simulink library "CryoDetLibCMB"  (R2016b)
settings: Solver=VariableStepAuto  StartTime=0.0  StopTime=10.0  RelTol=1e-3
values from neighbouring files (symbols this model uses):
  Fclk = Fadc    (= 307200000)    [setupCryoFPGA.m]    (also in setupCryoFPGA_CMB.m; setupCryoFPGAorig.m = 312500000)
undefined symbols (not defined in the file or in its folder): xlipgetpartsetting
libraries: xbsIndex_r4 x255, CryoDetLibCMB x19, CryoDetLib x2, simulink x1
(part 3 of 3)

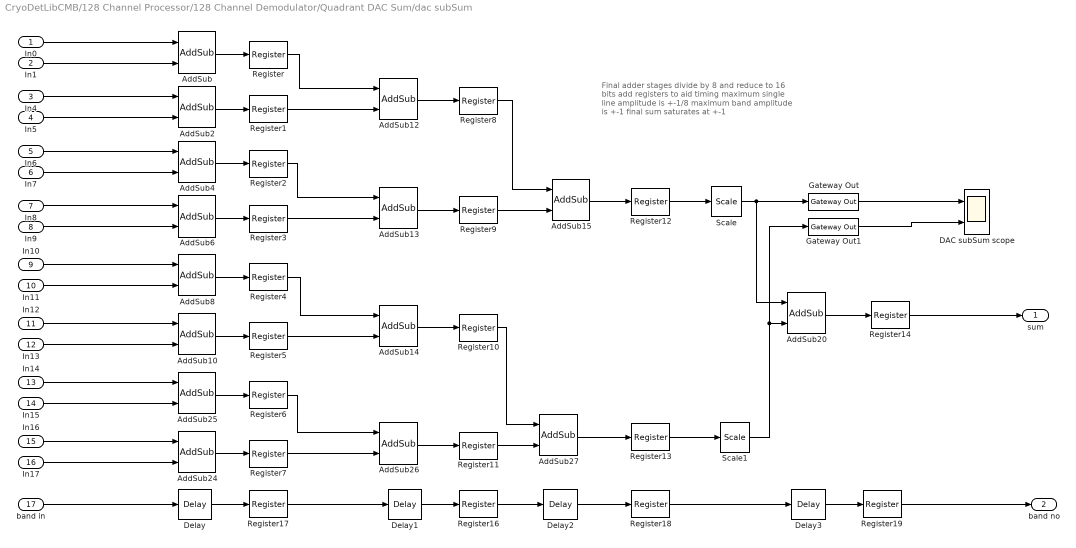
== system CryoDetLibCMB/128 Channel Processor/128 Channel Demodulator/Quadrant DAC Sum/dac subSum ==
  note: Final adder stages
      | divide by 8
      | and reduce to 16 bits
      | add registers to aid timing
      | maximum single line amplitude is +-1/8
      | maximum band amplitude is +-1
      | final sum saturates at +-1
  In0 : Inport
  In1 : Inport  Port=2
  In4 : Inport  Port=3
  In5 : Inport  Port=4
  In6 : Inport  Port=5
  In7 : Inport  Port=6
  In8 : Inport  Port=7
  In9 : Inport  Port=8
  In10 : Inport  Port=9
  In11 : Inport  Port=10
  In12 : Inport  Port=11
  In13 : Inport  Port=12
  In14 : Inport  Port=13
  In15 : Inport  Port=14
  In16 : Inport  Port=15
  In17 : Inport  Port=16
  band in : Inport  Port=17
  AddSub{,2,4,8,10,12..14,24..26} (11 alike) : xbsIndex_r4/AddSub  mode=Addition  use_carryin=off  use_carryout=off  en=off  latency=3  precision=User Defined  arith_type="Signed  (2's comp)"  n_bits=20  bin_pt=17  quantization=Truncate  overflow=Wrap  use_behavioral_HDL=off  hw_selection=Fabric  pipelined=off  dbl_ovrd=off  block_type=addsub
  AddSub15 : xbsIndex_r4/AddSub  mode=Addition  use_carryin=off  use_carryout=off  en=off  latency=3  precision=User Defined  arith_type="Signed  (2's comp)"  n_bits=21  bin_pt=17  quantization=Truncate  overflow=Wrap  use_behavioral_HDL=off  hw_selection=Fabric  pipelined=off  dbl_ovrd=off  block_type=addsub
  AddSub20 : xbsIndex_r4/AddSub  mode=Addition  use_carryin=off  use_carryout=off  en=off  latency=3  precision=User Defined  arith_type="Signed  (2's comp)"  n_bits=21  bin_pt=20  quantization=Truncate  overflow=Saturate  use_behavioral_HDL=off  hw_selection=Fabric  pipelined=off  dbl_ovrd=off  block_type=addsub
  AddSub27 : xbsIndex_r4/AddSub  mode=Addition  use_carryin=off  use_carryout=off  en=off  latency=3  precision=User Defined  arith_type="Signed  (2's comp)"  n_bits=21  bin_pt=17  quantization=Truncate  overflow=Wrap  use_behavioral_HDL=off  hw_selection=Fabric  pipelined=off  dbl_ovrd=off  block_type=addsub
  AddSub6 : xbsIndex_r4/AddSub  mode=Addition  use_carryin=off  use_carryout=off  en=off  latency=3  precision=User Defined  arith_type="Signed  (2's comp)"  n_bits=20  bin_pt=15  quantization=Truncate  overflow=Wrap  use_behavioral_HDL=off  hw_selection=Fabric  pipelined=off  dbl_ovrd=off  block_type=addsub
  DAC subSum scope : Scope  NumInputPorts=2
  Delay{,1..3} (4 alike) : xbsIndex_r4/Delay  rst=off  infoeditControl=Selection of Reset will increase slice count due to use of real FFs and instead of SRLs  en=off  latency=3  reg_retiming=on  dbl_ovrd=off  block_type=delay
  Gateway Out : xbsIndex_r4/Gateway Out  inherit_from_input=off  hdl_port=off  rows=1  columns=1  UseAsDAC=off  DACChannel='1'  interface=None  automatic_assignment=on  address_offset=hex2dec('00')  intf_name=''  intf_description=''  timing_constraint=None  locs_specified=off  LOCs={}  io_standard={}  block_type=gatewayout
  Gateway Out1 : xbsIndex_r4/Gateway Out  inherit_from_input=off  hdl_port=off  rows=1  columns=1  UseAsDAC=off  DACChannel='1'  interface=None  automatic_assignment=on  address_offset=hex2dec('00')  intf_name=''  intf_description=''  timing_constraint=None  locs_specified=off  LOCs={}  io_standard={}  block_type=gatewayout
  Register{,1..14,16..19} (19 alike) : xbsIndex_r4/Register  init=0  rst=off  en=off  dbl_ovrd=off  block_type=register
  Scale : xbsIndex_r4/Scale  scale_factor=-3  dbl_ovrd=off  block_type=scale
  Scale1 : xbsIndex_r4/Scale  scale_factor=-3  dbl_ovrd=off  block_type=scale
  sum : Outport
  band no : Outport  Port=2
  wires:
  Register14/1 -> sum/1
  Register13/1 -> Scale1/1
  Register12/1 -> Scale/1
  Register11/1 -> AddSub27/2
  Register10/1 -> AddSub27/1
  Register9/1 -> AddSub15/2
  Register8/1 -> AddSub15/1
  Register7/1 -> AddSub26/2
  Register6/1 -> AddSub26/1
  Register5/1 -> AddSub14/2
  Register4/1 -> AddSub14/1
  Register3/1 -> AddSub13/2
  Register2/1 -> AddSub13/1
  Register1/1 -> AddSub12/2
  Register/1 -> AddSub12/1
  Gateway Out/1 -> DAC subSum scope/1
  Gateway Out1/1 -> DAC subSum scope/2
  In9/1 -> AddSub6/2
  In1/1 -> AddSub/2
  In4/1 -> AddSub2/1
  In5/1 -> AddSub2/2
  In6/1 -> AddSub4/1
  In7/1 -> AddSub4/2
  In8/1 -> AddSub6/1
  In10/1 -> AddSub8/1
  In11/1 -> AddSub8/2
  In12/1 -> AddSub10/1
  In13/1 -> AddSub10/2
  In14/1 -> AddSub25/1
  In15/1 -> AddSub25/2
  In16/1 -> AddSub24/1
  In17/1 -> AddSub24/2
  AddSub26/1 -> Register11/1
  AddSub27/1 -> Register13/1
  AddSub14/1 -> Register10/1
  AddSub24/1 -> Register7/1
  AddSub25/1 -> Register6/1
  Scale1/1 -> AddSub20/2, Gateway Out1/1
  Scale/1 -> AddSub20/1, Gateway Out/1
  AddSub15/1 -> Register12/1
  AddSub13/1 -> Register9/1
  AddSub12/1 -> Register8/1
  AddSub10/1 -> Register5/1
  AddSub8/1 -> Register4/1
  AddSub6/1 -> Register3/1
  AddSub4/1 -> Register2/1
  AddSub2/1 -> Register1/1
  AddSub/1 -> Register/1
  AddSub20/1 -> Register14/1
  In0/1 -> AddSub/1
  Delay/1 -> Register17/1
  band in/1 -> Delay/1
  Register17/1 -> Delay1/1
  Delay1/1 -> Register16/1
  Register16/1 -> Delay2/1
  Delay2/1 -> Register18/1
  Register18/1 -> Delay3/1
  Delay3/1 -> Register19/1
  Register19/1 -> band no/1
